simulink model "OTHERSBEZIERMODEL"  (R2023a)
settings: Solver=FixedStepAuto  StartTime=0.0  StopTime=10.0  FixedStep=0.001  RelTol=1e-3
libraries: simulink_extras x4
settings Model: Creator=james  LastModifiedBy=james

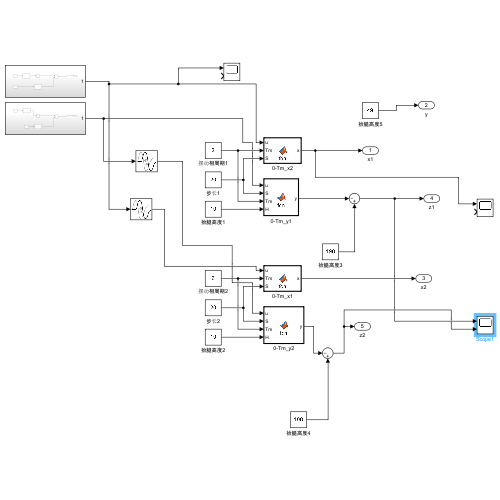
[thumbnail: Simulink's stored preview of the top-level diagram]
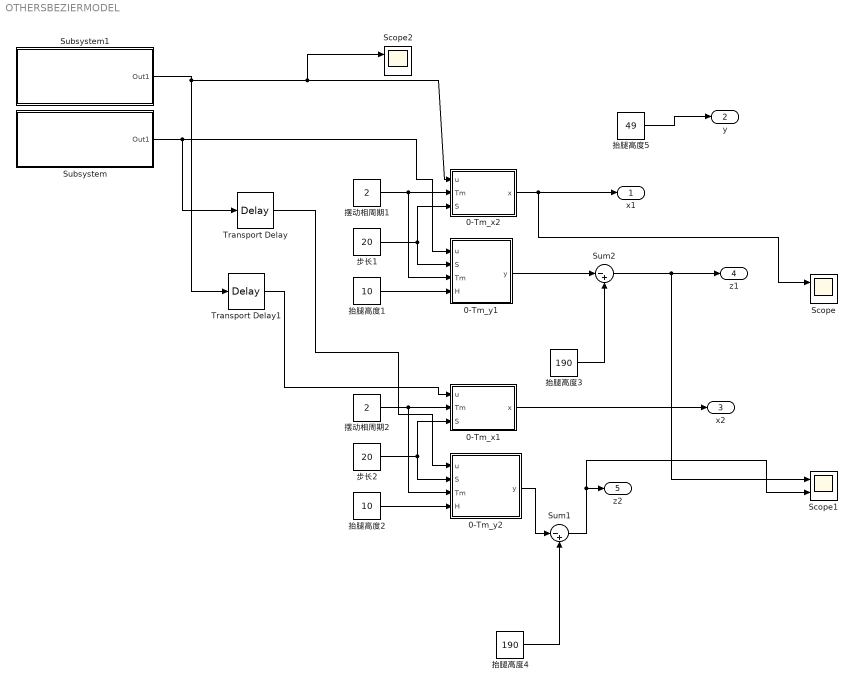
== system OTHERSBEZIERMODEL ==
  0-Tm_x1 : MATLAB Function  TreatAsAtomicUnit=on
  0-Tm_x2 : MATLAB Function  TreatAsAtomicUnit=on
  0-Tm_y1 : MATLAB Function  TreatAsAtomicUnit=on
  0-Tm_y2 : MATLAB Function  TreatAsAtomicUnit=on
  Scope : Scope  NumInputPorts=2
  Scope1 : Scope  NumInputPorts=2
  Scope2 : Scope  NumInputPorts=2
  Subsystem : Subsystem
  Subsystem1 : Subsystem
  Sum1 : Sum  Inputs=|-+
  Sum2 : Sum  Inputs=|-+
  Transport Delay : TransportDelay  DelayTime=2
  Transport Delay1 : TransportDelay  DelayTime=2
  抬腿高度1 : Constant  Value=10
  抬腿高度2 : Constant  Value=10
  抬腿高度3 : Constant  Value=190
  抬腿高度4 : Constant  Value=190
  抬腿高度5 : Constant  Value=49
  摆动相周期1 : Constant  Value=2
  摆动相周期2 : Constant  Value=2
  步长1 : Constant  Value=20
  步长2 : Constant  Value=20
  x1 : Outport  VectorParamsAs1DForOutWhenUnconnected=off
  y : Outport  Port=2  VectorParamsAs1DForOutWhenUnconnected=off
  x2 : Outport  Port=3  VectorParamsAs1DForOutWhenUnconnected=off
  z1 : Outport  Port=4  VectorParamsAs1DForOutWhenUnconnected=off
  z2 : Outport  Port=5  VectorParamsAs1DForOutWhenUnconnected=off
  wires:
  Transport Delay/1 -> 0-Tm_y2/1(u)
  0-Tm_y1/1(y) -> Sum2/1
  Sum2/1 -> Scope1/1, z1/1
  Sum1/1 -> Scope1/2, z2/1
  抬腿高度3/1 -> Sum2/2
  摆动相周期1/1 -> 0-Tm_y1/3(Tm), 0-Tm_x2/2(Tm)
  抬腿高度4/1 -> Sum1/2
  Transport Delay1/1 -> 0-Tm_x1/1(u)
  Subsystem1/1(Out1) -> Scope2/1, 0-Tm_x2/1(u), Transport Delay1/1
  0-Tm_y2/1(y) -> Sum1/1
  抬腿高度2/1 -> 0-Tm_y2/4(H)
  0-Tm_x1/1(x) -> x2/1
  Subsystem/1(Out1) -> 0-Tm_y1/1(u), Transport Delay/1
  步长1/1 -> 0-Tm_y1/2(S), 0-Tm_x2/3(S)
  抬腿高度5/1 -> y/1
  0-Tm_x2/1(x) -> Scope/1, x1/1
  步长2/1 -> 0-Tm_x1/3(S), 0-Tm_y2/2(S)
  摆动相周期2/1 -> 0-Tm_x1/2(Tm), 0-Tm_y2/3(Tm)
  抬腿高度1/1 -> 0-Tm_y1/4(H)

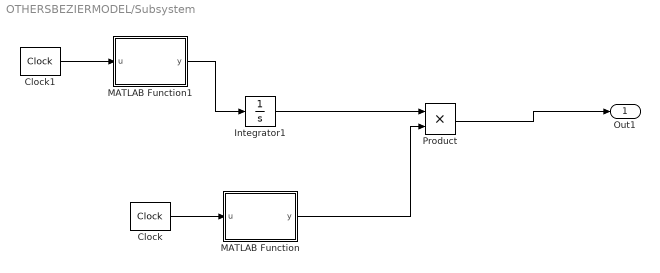
== system OTHERSBEZIERMODEL/Subsystem ==
  Clock : simulink_extras/Flip Flops/Clock  period=4
  Clock1 : simulink_extras/Flip Flops/Clock  period=2
  Integrator1 : Integrator
  MATLAB Function : MATLAB Function  TreatAsAtomicUnit=on
  MATLAB Function1 : MATLAB Function  TreatAsAtomicUnit=on
  Product : Product
  Out1 : Outport  VectorParamsAs1DForOutWhenUnconnected=off
  wires:
  MATLAB Function1/1(y) -> Integrator1/1
  Clock1/1 -> MATLAB Function1/1(u)
  MATLAB Function/1(y) -> Product/2
  Clock/1 -> MATLAB Function/1(u)
  Integrator1/1 -> Product/1
  Product/1 -> Out1/1

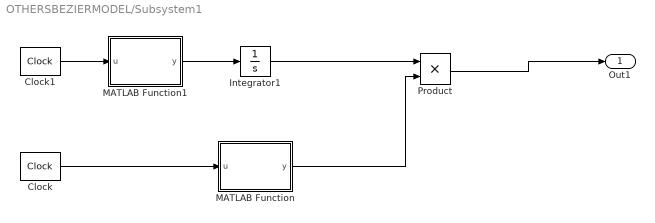
== system OTHERSBEZIERMODEL/Subsystem1 ==
  Clock : simulink_extras/Flip Flops/Clock  period=8
  Clock1 : simulink_extras/Flip Flops/Clock  period=4
  Integrator1 : Integrator
  MATLAB Function : MATLAB Function  TreatAsAtomicUnit=on
  MATLAB Function1 : MATLAB Function  TreatAsAtomicUnit=on
  Product : Product
  Out1 : Outport  VectorParamsAs1DForOutWhenUnconnected=off
  wires:
  MATLAB Function1/1(y) -> Integrator1/1
  Clock1/1 -> MATLAB Function1/1(u)
  MATLAB Function/1(y) -> Product/2
  Clock/1 -> MATLAB Function/1(u)
  Integrator1/1 -> Product/1
  Product/1 -> Out1/1

== matlab function OTHERSBEZIERMODEL/0-Tm_x1 ==
  data: u input; x output; Tm input; S input
function x = fcn(u,Tm,S)


if u>0
   
    x =S*(u/Tm-1/(2*pi)*sin(2*pi*u/Tm));
else 
    u=-u;
    x =S*(u/Tm-1/(2*pi)*sin(2*pi*u/Tm));
end

== matlab function OTHERSBEZIERMODEL/0-Tm_y1 ==
  data: u input; y output; S input; Tm input; H input
function y = fcn(u,S,Tm,H)

n=4;
if u>0
    y=2*H*(u/Tm-1/(n*pi)*sin(n*pi*u/Tm)).*(u>=0&u<Tm/2)+2*H*(1-u/Tm+1/(n*pi)*sin(n*pi*u/Tm)).*(u>=Tm/2&u<Tm);;
else 
    y=0;
end

== matlab function OTHERSBEZIERMODEL/0-Tm_x2 ==
  data: u input; x output; Tm input; S input
function x = fcn(u,Tm,S)

if u>0
    x =S*(u/Tm-1/(2*pi)*sin(2*pi*u/Tm));
else 
    u=-u;
     x =S*(u/Tm-1/(2*pi)*sin(2*pi*u/Tm));
end

== matlab function OTHERSBEZIERMODEL/0-Tm_y2 ==
  data: u input; y output; S input; Tm input; H input
function y = fcn(u,S,Tm,H)

n=4;
if u>0
    y=2*H*(u/Tm-1/(n*pi)*sin(n*pi*u/Tm)).*(u>=0&u<Tm/2)+2*H*(1-u/Tm+1/(n*pi)*sin(n*pi*u/Tm)).*(u>=Tm/2&u<Tm);;
else 
    y=0;
end

== matlab function OTHERSBEZIERMODEL/Subsystem/MATLAB Function ==
  data: u input; y output
function y = fcn(u)
if u==0
    y = -1;
else
    y=1;
end
end

== matlab function OTHERSBEZIERMODEL/Subsystem/MATLAB Function1 ==
  data: u input; y output
function y = fcn(u)
if u==0
    y = -1;
else
    y=1;
end
end

== matlab function OTHERSBEZIERMODEL/Subsystem1/MATLAB Function ==
  data: u input; y output
function y = fcn(u)
if u==0
    y = -1;
else
    y=1;
end
end

== matlab function OTHERSBEZIERMODEL/Subsystem1/MATLAB Function1 ==
  data: u input; y output
function y = fcn(u)
if u==0
    y = -1;
else
    y=1;
end
end
